simulink model "RecvL4sStEnCtrl"  (R2018b)
settings: Solver=FixedStepDiscrete  StartTime=0.0  StopTime=10.0  FixedStep=0.01  RelTol=1e-3
undefined symbols (not defined in the file or in its folder): data, KeSMSw4SSecRwLtStLgrstOtwdInwdClosePos1_Val, KeSMSw4SSecRwLtStLgrstUpwdDnwdClosePos1_Val, KeSMSw4SSecRwLtStLgrstUpwdDnwdClosePos2_Val, SecRwLtStBkReclnEn_Clear, SecRwLtStBkReclnEn_Set, SecRwLtStFtrstEn_Clear, SecRwLtStFtrstEn_Set, SecRwLtStHdrstFwdBkwdEn_Clear, SecRwLtStHdrstFwdBkwdEn_Set, SecRwLtStHdrstUpwdDnwdEn_Clear, SecRwLtStHdrstUpwdDnwdEn_Set, SecRwLtStLgrstInwdOtwdEn_Clear, SecRwLtStLgrstInwdOtwdEn_Set, SecRwLtStLgrstUpwdDnwdEn_Clear, SecRwLtStLgrstUpwdDnwdEn_Set
libraries: simulink x13
settings Model: Creator=sn2xws  LastModifiedBy=sn2xws
settings DataIOCC: SaveFormat=StructureWithTime
settings OptimizationCC: DefaultParameterBehavior=Inlined  EnhancedBackFolding=on  PassReuseOutputArgsAs=Individual arguments  ZeroExternalMemoryAtStartup=off  ZeroInternalMemoryAtStartup=off  OptimizeBlockOrder=speed  DifferentSizesBufferReuse=on  OptimizationCustomize=off
settings DebuggingCC: ParameterTunabilityLossMsg=error
settings SFSimCC: MATLABDynamicMemAlloc=off
settings RTWCC: SystemTargetFile=autosar.tlc  GenCodeOnly=on  TemplateMakefile=ert_default_tmf  Description=AUTOSAR  GenerateReport=on  IncludeHyperlinkInReport=on  LaunchReport=on  GenerateTraceInfo=on  GenerateTraceReport=on  GenerateTraceReportSl=on  GenerateTraceReportSf=on  GenerateTraceReportEml=on  GenerateCodeMetricsReport=on
settings CodeAppCC: ForceParamTrailComments=on  IgnoreCustomStorageClasses=off  OperatorAnnotations=on  SimulinkDataObjDesc=on  SFDataObjDesc=on  InsertBlockDesc=on
settings STFCustomTargetCC: TargetLangStandard=C99 (ISO)  MultiwordLength=256  ParMdlRefBuildCompliant=on  CompOptLevelCompliant=on  IncludeMdlTerminateFcn=off  CombineOutputUpdateFcns=on  SuppressErrorStatus=on  ERTCustomFileBanners=on  SupportNonFinite=off  SupportComplex=off  SupportContinuousTime=off  SupportNonInlinedSFcns=off  RemoveResetFunc=on  MATLABClassNameForMDSCustomization=Simulink.SoftwareTarget.ERTCustomization  AutosarCompliant=on  UseToolchainInfoCompliant=on  LookupTableObjectStructAxisOrder=2,1,3,4,...  LUTObjectStructOrderEvenSpacing=Size,Table,Breakpoints  SystemTargetFile=autosar.tlc
settings ERTTargetCC: TargetLangStandard=C99 (ISO)  ConcurrentExecutionCompliant=off  IncludeMdlTerminateFcn=off  SuppressErrorStatus=on  SupportNonFinite=off  SupportComplex=off  ModelStepFunctionPrototypeControlCompliant=off  CPPClassGenCompliant=off  AutosarCompliant=on  LookupTableObjectStructAxisOrder=2,1,3,4,...  LUTObjectStructOrderEvenSpacing=Size,Table,Breakpoints  InlinedParameterPlacement=NonHierarchical  ERTCustomFileTemplate=example_file_process.tlc  ERTFilePackagingFormat=Compact

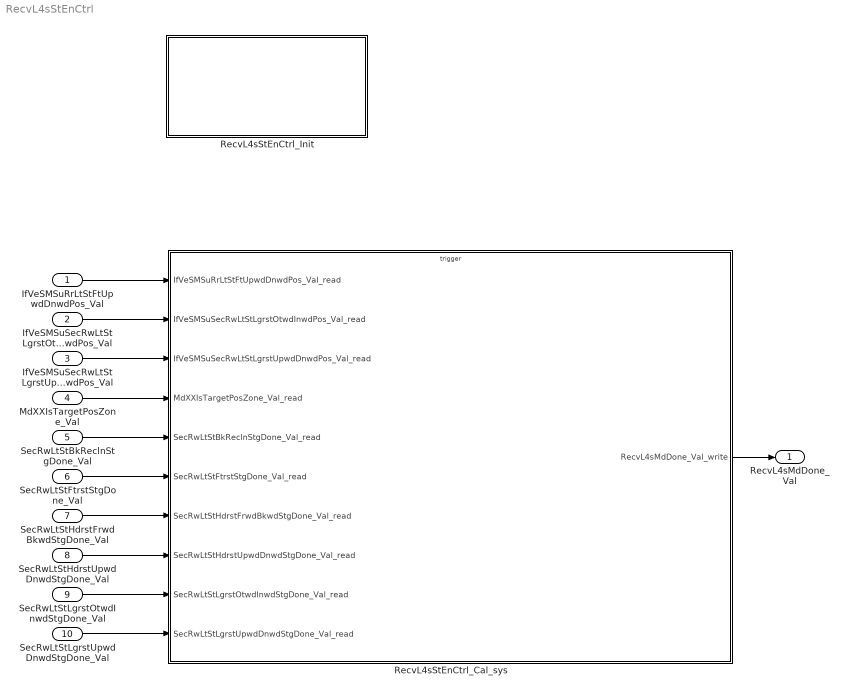
== system RecvL4sStEnCtrl ==
  IfVeSMSuRrLtStFtUpwdDnwdPos_Val : Inport  OutDataTypeStr=uint16  PortDimensions=1
  IfVeSMSuSecRwLtStLgrstOtwdInwdPos_Val : Inport  Port=2  OutDataTypeStr=uint16  PortDimensions=1
  IfVeSMSuSecRwLtStLgrstUpwdDnwdPos_Val : Inport  Port=3  OutDataTypeStr=uint16  PortDimensions=1
  MdXXIsTargetPosZone_Val : Inport  Port=4  OutDataTypeStr=uint32  PortDimensions=1
  SecRwLtStBkReclnStgDone_Val : Inport  Port=5  OutDataTypeStr=boolean  PortDimensions=1
  SecRwLtStFtrstStgDone_Val : Inport  Port=6  OutDataTypeStr=boolean  PortDimensions=1
  SecRwLtStHdrstFrwdBkwdStgDone_Val : Inport  Port=7  OutDataTypeStr=boolean  PortDimensions=1
  SecRwLtStHdrstUpwdDnwdStgDone_Val : Inport  Port=8  OutDataTypeStr=boolean  PortDimensions=1
  SecRwLtStLgrstOtwdInwdStgDone_Val : Inport  Port=9  OutDataTypeStr=boolean  PortDimensions=1
  SecRwLtStLgrstUpwdDnwdStgDone_Val : Inport  Port=10  OutDataTypeStr=boolean  PortDimensions=1
  RecvL4sStEnCtrl_Cal_sys : Subsystem
  RecvL4sStEnCtrl_Init : Subsystem
  RecvL4sMdDone_Val : Outport  OutDataTypeStr=uint8  PortDimensions=1
  wires:
  IfVeSMSuRrLtStFtUpwdDnwdPos_Val/1 -> RecvL4sStEnCtrl_Cal_sys/1(IfVeSMSuRrLtStFtUpwdDnwdPos_Val_read)
  IfVeSMSuSecRwLtStLgrstOtwdInwdPos_Val/1 -> RecvL4sStEnCtrl_Cal_sys/2(IfVeSMSuSecRwLtStLgrstOtwdInwdPos_Val_read)
  IfVeSMSuSecRwLtStLgrstUpwdDnwdPos_Val/1 -> RecvL4sStEnCtrl_Cal_sys/3(IfVeSMSuSecRwLtStLgrstUpwdDnwdPos_Val_read)
  MdXXIsTargetPosZone_Val/1 -> RecvL4sStEnCtrl_Cal_sys/4(MdXXIsTargetPosZone_Val_read)
  SecRwLtStBkReclnStgDone_Val/1 -> RecvL4sStEnCtrl_Cal_sys/5(SecRwLtStBkReclnStgDone_Val_read)
  SecRwLtStFtrstStgDone_Val/1 -> RecvL4sStEnCtrl_Cal_sys/6(SecRwLtStFtrstStgDone_Val_read)
  SecRwLtStHdrstFrwdBkwdStgDone_Val/1 -> RecvL4sStEnCtrl_Cal_sys/7(SecRwLtStHdrstFrwdBkwdStgDone_Val_read)
  SecRwLtStHdrstUpwdDnwdStgDone_Val/1 -> RecvL4sStEnCtrl_Cal_sys/8(SecRwLtStHdrstUpwdDnwdStgDone_Val_read)
  SecRwLtStLgrstOtwdInwdStgDone_Val/1 -> RecvL4sStEnCtrl_Cal_sys/9(SecRwLtStLgrstOtwdInwdStgDone_Val_read)
  SecRwLtStLgrstUpwdDnwdStgDone_Val/1 -> RecvL4sStEnCtrl_Cal_sys/10(SecRwLtStLgrstUpwdDnwdStgDone_Val_read)
  RecvL4sStEnCtrl_Cal_sys/1(RecvL4sMdDone_Val_write) -> RecvL4sMdDone_Val/1

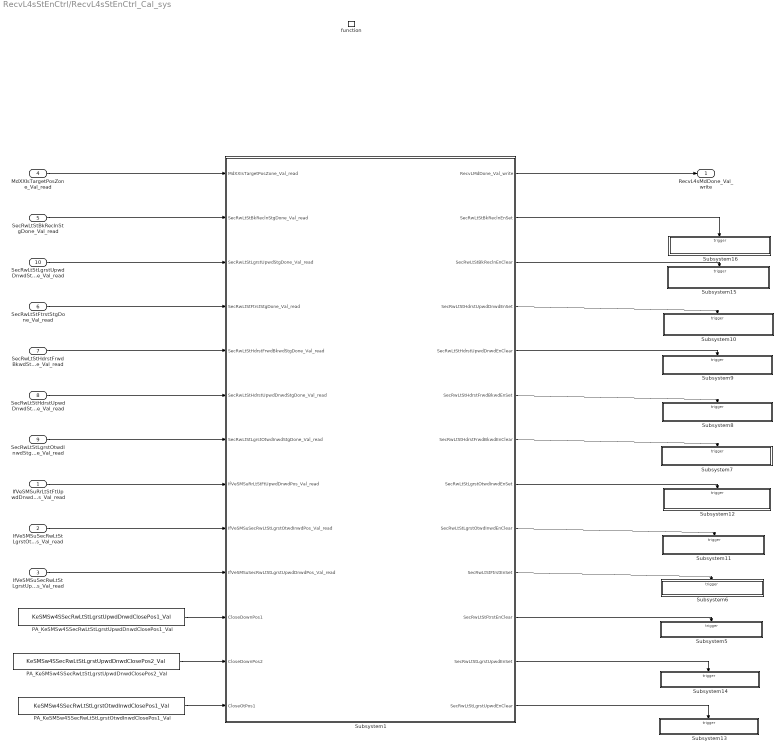
== system RecvL4sStEnCtrl/RecvL4sStEnCtrl_Cal_sys ==
  IfVeSMSuRrLtStFtUpwdDnwdPos_Val_read : Inport
  IfVeSMSuSecRwLtStLgrstOtwdInwdPos_Val_read : Inport  Port=2
  IfVeSMSuSecRwLtStLgrstUpwdDnwdPos_Val_read : Inport  Port=3
  MdXXIsTargetPosZone_Val_read : Inport  Port=4
  SecRwLtStBkReclnStgDone_Val_read : Inport  Port=5
  SecRwLtStFtrstStgDone_Val_read : Inport  Port=6
  SecRwLtStHdrstFrwdBkwdStgDone_Val_read : Inport  Port=7
  SecRwLtStHdrstUpwdDnwdStgDone_Val_read : Inport  Port=8
  SecRwLtStLgrstOtwdInwdStgDone_Val_read : Inport  Port=9
  SecRwLtStLgrstUpwdDnwdStgDone_Val_read : Inport  Port=10
  function : TriggerPort  TriggerType=function-call  IsSimulinkFunction=on  FunctionName=RecvL4sStEnCtrl_Cal  VariantControl=(inherit)
  PA_KeSMSw4SSecRwLtStLgrstOtwdInwdClosePos1_Val : Constant  Value=KeSMSw4SSecRwLtStLgrstOtwdInwdClosePos1_Val
  PA_KeSMSw4SSecRwLtStLgrstUpwdDnwdClosePos1_Val : Constant  Value=KeSMSw4SSecRwLtStLgrstUpwdDnwdClosePos1_Val
  PA_KeSMSw4SSecRwLtStLgrstUpwdDnwdClosePos2_Val : Constant  Value=KeSMSw4SSecRwLtStLgrstUpwdDnwdClosePos2_Val
  Subsystem1 : Subsystem
  Subsystem10 : Subsystem
  Subsystem11 : Subsystem
  Subsystem12 : Subsystem
  Subsystem13 : Subsystem
  Subsystem14 : Subsystem
  Subsystem15 : Subsystem
  Subsystem16 : Subsystem
  Subsystem5 : Subsystem
  Subsystem6 : Subsystem
  Subsystem7 : Subsystem
  Subsystem8 : Subsystem
  Subsystem9 : Subsystem
  RecvL4sMdDone_Val_write : Outport
      settings: EnsureOutportIsVirtual=on
  wires:
  SecRwLtStHdrstFrwdBkwdStgDone_Val_read/1 -> Subsystem1/5(SecRwLtStHdrstFrwdBkwdStgDone_Val_read)
  MdXXIsTargetPosZone_Val_read/1 -> Subsystem1/1(MdXXIsTargetPosZone_Val_read)
  SecRwLtStBkReclnStgDone_Val_read/1 -> Subsystem1/2(SecRwLtStBkReclnStgDone_Val_read)
  SecRwLtStLgrstUpwdDnwdStgDone_Val_read/1 -> Subsystem1/3(SecRwLtStLgrstUpwdStgDone_Val_read)
  SecRwLtStFtrstStgDone_Val_read/1 -> Subsystem1/4(SecRwLtStFtrstStgDone_Val_read)
  SecRwLtStHdrstUpwdDnwdStgDone_Val_read/1 -> Subsystem1/6(SecRwLtStHdrstUpwdDnwdStgDone_Val_read)
  SecRwLtStLgrstOtwdInwdStgDone_Val_read/1 -> Subsystem1/7(SecRwLtStLgrstOtwdInwdStgDone_Val_read)
  IfVeSMSuRrLtStFtUpwdDnwdPos_Val_read/1 -> Subsystem1/8(IfVeSMSuRrLtStFtUpwdDnwdPos_Val_read)
  IfVeSMSuSecRwLtStLgrstOtwdInwdPos_Val_read/1 -> Subsystem1/9(IfVeSMSuSecRwLtStLgrstOtwdInwdPos_Val_read)
  IfVeSMSuSecRwLtStLgrstUpwdDnwdPos_Val_read/1 -> Subsystem1/10(IfVeSMSuSecRwLtStLgrstUpwdDnwdPos_Val_read)
  PA_KeSMSw4SSecRwLtStLgrstOtwdInwdClosePos1_Val/1 -> Subsystem1/13(CloseOtPos1)
  PA_KeSMSw4SSecRwLtStLgrstUpwdDnwdClosePos1_Val/1 -> Subsystem1/11(CloseDownPos1)
  PA_KeSMSw4SSecRwLtStLgrstUpwdDnwdClosePos2_Val/1 -> Subsystem1/12(CloseDownPos2)
  Subsystem1/1(RecvLMdDone_Val_write) -> RecvL4sMdDone_Val_write/1
  Subsystem1/5(SecRwLtStHdrstUpwdDnwdEnClear) -> Subsystem9/Trigger
  Subsystem1/3(SecRwLtStBkReclnEnClear) -> Subsystem15/Trigger
  Subsystem1/9(SecRwLtStLgrstOtwdInwdEnClear) -> Subsystem11/Trigger
  Subsystem1/8(SecRwLtStLgrstOtwdInwdEnSet) -> Subsystem12/Trigger
  Subsystem1/6(SecRwLtStHdrstFrwdBkwdEnSet) -> Subsystem8/Trigger
  Subsystem1/12(SecRwLtStLgrstUpwdEnSet) -> Subsystem14/Trigger
  Subsystem1/13(SecRwLtStLgrstUpwdEnClear) -> Subsystem13/Trigger
  Subsystem1/2(SecRwLtStBkReclnEnSet) -> Subsystem16/Trigger
  Subsystem1/11(SecRwLtStFtrstEnClear) -> Subsystem5/Trigger
  Subsystem1/7(SecRwLtStHdrstFrwdBkwdEnClear) -> Subsystem7/Trigger
  Subsystem1/10(SecRwLtStFtrstEnSet) -> Subsystem6/Trigger
  Subsystem1/4(SecRwLtStHdrstUpwdDnwdEnSet) -> Subsystem10/Trigger

== system RecvL4sStEnCtrl/RecvL4sStEnCtrl_Init ==
  Event Listener : EventListener  EventName=reset

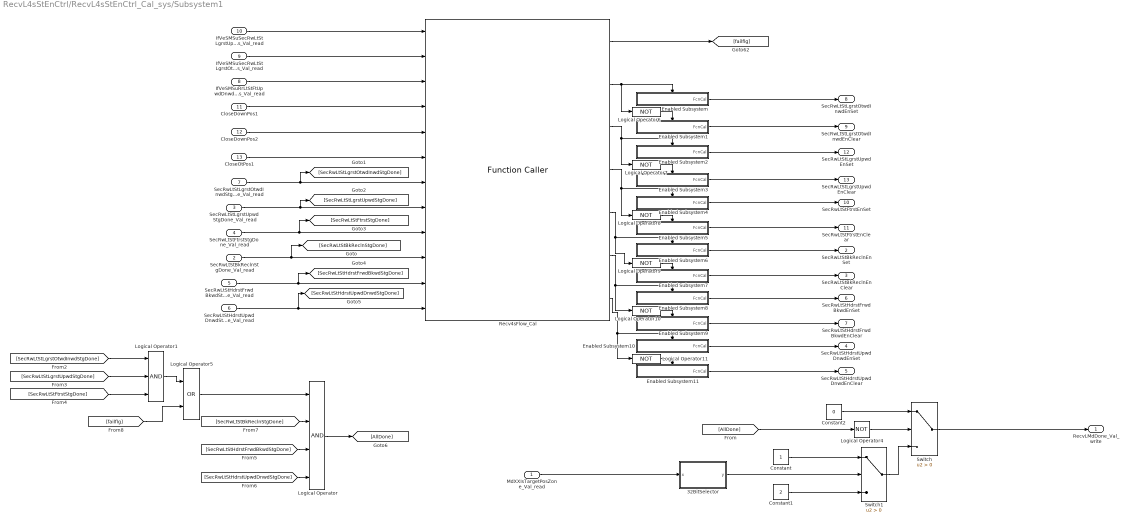
== system RecvL4sStEnCtrl/RecvL4sStEnCtrl_Cal_sys/Subsystem1 ==
  MdXXIsTargetPosZone_Val_read : Inport
  SecRwLtStBkReclnStgDone_Val_read : Inport  Port=2
  SecRwLtStLgrstUpwdStgDone_Val_read : Inport  Port=3
  SecRwLtStFtrstStgDone_Val_read : Inport  Port=4
  SecRwLtStHdrstFrwdBkwdStgDone_Val_read : Inport  Port=5
  SecRwLtStHdrstUpwdDnwdStgDone_Val_read : Inport  Port=6
  SecRwLtStLgrstOtwdInwdStgDone_Val_read : Inport  Port=7
  IfVeSMSuRrLtStFtUpwdDnwdPos_Val_read : Inport  Port=8
  IfVeSMSuSecRwLtStLgrstOtwdInwdPos_Val_read : Inport  Port=9
  IfVeSMSuSecRwLtStLgrstUpwdDnwdPos_Val_read : Inport  Port=10
  CloseDownPos1 : Inport  Port=11
  CloseDownPos2 : Inport  Port=12
  CloseOtPos1 : Inport  Port=13
  32BitSelector : Subsystem  mask(32 Bit Selector){BitNum=10}
      mask prompts: BitNum "Select Bit Number"
      mask help: Allows selection of a particular bit (0-31) out of a packed word up to 32 bits long. Output will be true if the bit number selected via the mask parameter is equal to one.
      mask TypeOptions BitNum: 0 | 1 | 2 | 3 | 4 | 5 | 6 | 7 | 8 | 9 | 10 | 11 | 12 | 13 | 14 | 15 | 16 | 17 | 18 | 19 | 20 | 21 | 22 | 23 | 24 | 25 | 26 | 27 | 28 | 29 | 30 | 31
      mask Display:
      | text(0.5, 0.8,'BIT','horizontalAlignment','center')
      | text(0.5, 0.5,'SELECTOR','horizontalAlignment','center')
      | text(0.5, 0.2,['-- Bit ',char(get_param(gcb,'BitNum')),' --'],'horizontalAlignment','center')
  Constant : Constant  OutDataTypeStr=uint8
  Constant1 : Constant  Value=2  OutDataTypeStr=uint8
  Constant2 : Constant  Value=0  OutDataTypeStr=uint8
  Enabled Subsystem : Subsystem  TreatAsAtomicUnit=on
  Enabled Subsystem1 : Subsystem  TreatAsAtomicUnit=on
  Enabled Subsystem10 : Subsystem  TreatAsAtomicUnit=on
  Enabled Subsystem11 : Subsystem  TreatAsAtomicUnit=on
  Enabled Subsystem2 : Subsystem  TreatAsAtomicUnit=on
  Enabled Subsystem3 : Subsystem  TreatAsAtomicUnit=on
  Enabled Subsystem4 : Subsystem  TreatAsAtomicUnit=on
  Enabled Subsystem5 : Subsystem  TreatAsAtomicUnit=on
  Enabled Subsystem6 : Subsystem  TreatAsAtomicUnit=on
  Enabled Subsystem7 : Subsystem  TreatAsAtomicUnit=on
  Enabled Subsystem8 : Subsystem  TreatAsAtomicUnit=on
  Enabled Subsystem9 : Subsystem  TreatAsAtomicUnit=on
  Logical Operator : Logic  Inputs=4  AllPortsSameDT=off  OutDataTypeStr=boolean
  Logical Operator1 : Logic  Inputs=3  AllPortsSameDT=off  OutDataTypeStr=boolean
  Logical Operator{4,6..11} (7 alike) : Logic  Operator=NOT  AllPortsSameDT=off  OutDataTypeStr=boolean
  Logical Operator5 : Logic  Operator=OR  AllPortsSameDT=off  OutDataTypeStr=boolean
  Recv4sFlow_Cal : FunctionCaller  FunctionPrototype=[Failflg,LgrstInwdOtwdEn,LgrstUpwdDnwdEn,FtrstEn,BkReclnEn,HdrstFrwdBkwdEn,HdrstUpwdDnwdEn] = Recv4sFlow_Cal(LgrstUpwdDnwdPos,LgrstOtwdInwdPos,FtUpwdDnwdPos,CloseDnwdPos1,CloseDnwdPos2,CloseOtwdPos1,LgrstInwdStgDone,LgrstUpwdStgDone,FtrstStgDone,BkReclnStgDone,HdrstFwdBkwdStgDone,HdrstupwdDnwdStgDone)  InputArgumentSpecifications=uint16(1), uint16(1), uint16(1), uint16(1), uint16(1), uint16(1), boolean(true), boolean(true), boolean(true), boolean(true), boolean(true), boolean(true)  OutputArgumentSpecifications=boolean(true), boolean(true), boolean(true), boolean(true), boolean(true), boolean(true), boolean(true)
  Switch : Switch  Criteria=u2 > Threshold
  Switch1 : Switch  Criteria=u2 > Threshold
  RecvLMdDone_Val_write : Outport
      settings: EnsureOutportIsVirtual=on
  SecRwLtStBkReclnEnSet : Outport  Port=2
  SecRwLtStBkReclnEnClear : Outport  Port=3
  SecRwLtStHdrstUpwdDnwdEnSet : Outport  Port=4
  SecRwLtStHdrstUpwdDnwdEnClear : Outport  Port=5
  SecRwLtStHdrstFrwdBkwdEnSet : Outport  Port=6
  SecRwLtStHdrstFrwdBkwdEnClear : Outport  Port=7
  SecRwLtStLgrstOtwdInwdEnSet : Outport  Port=8
  SecRwLtStLgrstOtwdInwdEnClear : Outport  Port=9
  SecRwLtStFtrstEnSet : Outport  Port=10
  SecRwLtStFtrstEnClear : Outport  Port=11
  SecRwLtStLgrstUpwdEnSet : Outport  Port=12
  SecRwLtStLgrstUpwdEnClear : Outport  Port=13
  wires:
  SecRwLtStLgrstOtwdInwdStgDone_Val_read/1 -> Recv4sFlow_Cal/7, [SecRwLtStLgrstOtwdInwdStgDone]
  Recv4sFlow_Cal/1 -> [failflg]
  CloseDownPos2/1 -> Recv4sFlow_Cal/5
  SecRwLtStHdrstUpwdDnwdStgDone_Val_read/1 -> [SecRwLtStHdrstUpwdDnwdStgDone], Recv4sFlow_Cal/12
  IfVeSMSuRrLtStFtUpwdDnwdPos_Val_read/1 -> Recv4sFlow_Cal/3
  CloseDownPos1/1 -> Recv4sFlow_Cal/4
  SecRwLtStHdrstFrwdBkwdStgDone_Val_read/1 -> [SecRwLtStHdrstFrwdBkwdStgDone], Recv4sFlow_Cal/11
  CloseOtPos1/1 -> Recv4sFlow_Cal/6
  IfVeSMSuSecRwLtStLgrstUpwdDnwdPos_Val_read/1 -> Recv4sFlow_Cal/1
  SecRwLtStBkReclnStgDone_Val_read/1 -> [SecRwLtStBkReclnStgDone], Recv4sFlow_Cal/10
  IfVeSMSuSecRwLtStLgrstOtwdInwdPos_Val_read/1 -> Recv4sFlow_Cal/2
  SecRwLtStLgrstUpwdStgDone_Val_read/1 -> Recv4sFlow_Cal/8, [SecRwLtStLgrstUpwdStgDone]
  Switch/1 -> RecvLMdDone_Val_write/1
  MdXXIsTargetPosZone_Val_read/1 -> 32BitSelector/1(x)
  Switch1/1 -> Switch/3
  SecRwLtStFtrstStgDone_Val_read/1 -> [SecRwLtStFtrstStgDone], Recv4sFlow_Cal/9
  Logical Operator5/1 -> Logical Operator/1
  [SecRwLtStFtrstStgDone] -> Logical Operator1/3
  Logical Operator1/1 -> Logical Operator5/1
  [SecRwLtStLgrstOtwdInwdStgDone] -> Logical Operator1/1
  [failflg] -> Logical Operator5/2
  [SecRwLtStLgrstUpwdStgDone] -> Logical Operator1/2
  [SecRwLtStHdrstUpwdDnwdStgDone] -> Logical Operator/4
  [SecRwLtStHdrstFrwdBkwdStgDone] -> Logical Operator/3
  [SecRwLtStBkReclnStgDone] -> Logical Operator/2
  Logical Operator/1 -> [AllDone]
  Enabled Subsystem6/1(FcnCal) -> SecRwLtStBkReclnEnSet/1
  Enabled Subsystem7/1(FcnCal) -> SecRwLtStBkReclnEnClear/1
  Enabled Subsystem2/1(FcnCal) -> SecRwLtStLgrstUpwdEnSet/1
  Enabled Subsystem3/1(FcnCal) -> SecRwLtStLgrstUpwdEnClear/1
  Enabled Subsystem10/1(FcnCal) -> SecRwLtStHdrstUpwdDnwdEnSet/1
  Enabled Subsystem11/1(FcnCal) -> SecRwLtStHdrstUpwdDnwdEnClear/1
  Enabled Subsystem8/1(FcnCal) -> SecRwLtStHdrstFrwdBkwdEnSet/1
  Enabled Subsystem9/1(FcnCal) -> SecRwLtStHdrstFrwdBkwdEnClear/1
  Enabled Subsystem/1(FcnCal) -> SecRwLtStLgrstOtwdInwdEnSet/1
  Enabled Subsystem1/1(FcnCal) -> SecRwLtStLgrstOtwdInwdEnClear/1
  Recv4sFlow_Cal/2 -> Logical Operator6/1, Enabled Subsystem/Enable
  Logical Operator6/1 -> Enabled Subsystem1/Enable
  Logical Operator7/1 -> Enabled Subsystem3/Enable
  Recv4sFlow_Cal/3 -> Logical Operator7/1, Enabled Subsystem2/Enable
  Recv4sFlow_Cal/4 -> Enabled Subsystem4/Enable, Logical Operator8/1
  Logical Operator8/1 -> Enabled Subsystem5/Enable
  Enabled Subsystem4/1(FcnCal) -> SecRwLtStFtrstEnSet/1
  Enabled Subsystem5/1(FcnCal) -> SecRwLtStFtrstEnClear/1
  Logical Operator9/1 -> Enabled Subsystem7/Enable
  Recv4sFlow_Cal/5 -> Enabled Subsystem6/Enable, Logical Operator9/1
  Recv4sFlow_Cal/6 -> Enabled Subsystem8/Enable, Logical Operator10/1
  Logical Operator10/1 -> Enabled Subsystem9/Enable
  Logical Operator11/1 -> Enabled Subsystem11/Enable
  Recv4sFlow_Cal/7 -> Logical Operator11/1, Enabled Subsystem10/Enable
  Constant2/1 -> Switch/1
  Constant1/1 -> Switch1/3
  Constant/1 -> Switch1/1
  [AllDone] -> Logical Operator4/1
  Logical Operator4/1 -> Switch/2
  32BitSelector/1(y) -> Switch1/2

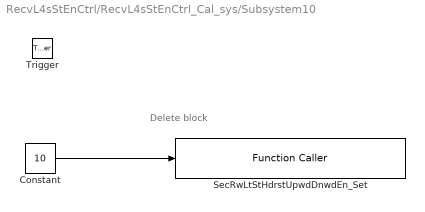
== system RecvL4sStEnCtrl/RecvL4sStEnCtrl_Cal_sys/Subsystem10 ==
  note: Delete block
  Trigger : TriggerPort  TriggerType=function-call  VariantControl=Variant  PortDimensions=1
  Constant : Constant  Value=10  OutDataTypeStr=uint8
  SecRwLtStHdrstUpwdDnwdEn_Set : FunctionCaller  FunctionPrototype=SecRwLtStHdrstUpwdDnwdEn_Set(data)  InputArgumentSpecifications=uint8(1)
  wires:
  Constant/1 -> SecRwLtStHdrstUpwdDnwdEn_Set/1

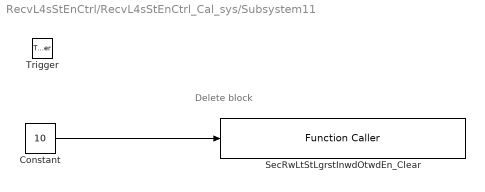
== system RecvL4sStEnCtrl/RecvL4sStEnCtrl_Cal_sys/Subsystem11 ==
  note: Delete block
  Trigger : TriggerPort  TriggerType=function-call  VariantControl=Variant  PortDimensions=1
  Constant : Constant  Value=10  OutDataTypeStr=uint8
  SecRwLtStLgrstInwdOtwdEn_Clear : FunctionCaller  FunctionPrototype=SecRwLtStLgrstInwdOtwdEn_Clear(data)  InputArgumentSpecifications=uint8(1)
  wires:
  Constant/1 -> SecRwLtStLgrstInwdOtwdEn_Clear/1

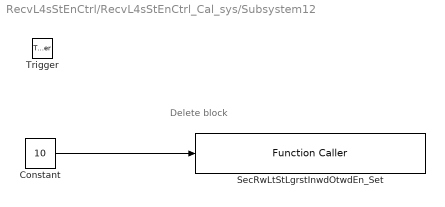
== system RecvL4sStEnCtrl/RecvL4sStEnCtrl_Cal_sys/Subsystem12 ==
  note: Delete block
  Trigger : TriggerPort  TriggerType=function-call  VariantControl=Variant  PortDimensions=1
  Constant : Constant  Value=10  OutDataTypeStr=uint8
  SecRwLtStLgrstInwdOtwdEn_Set : FunctionCaller  FunctionPrototype=SecRwLtStLgrstInwdOtwdEn_Set(data)  InputArgumentSpecifications=uint8(1)
  wires:
  Constant/1 -> SecRwLtStLgrstInwdOtwdEn_Set/1

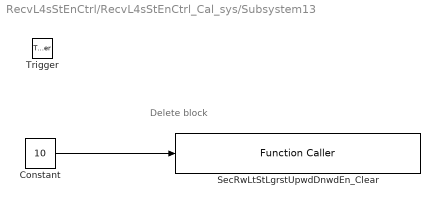
== system RecvL4sStEnCtrl/RecvL4sStEnCtrl_Cal_sys/Subsystem13 ==
  note: Delete block
  Trigger : TriggerPort  TriggerType=function-call  VariantControl=Variant  PortDimensions=1
  Constant : Constant  Value=10  OutDataTypeStr=uint8
  SecRwLtStLgrstUpwdDnwdEn_Clear : FunctionCaller  FunctionPrototype=SecRwLtStLgrstUpwdDnwdEn_Clear(data)  InputArgumentSpecifications=uint8(1)
  wires:
  Constant/1 -> SecRwLtStLgrstUpwdDnwdEn_Clear/1

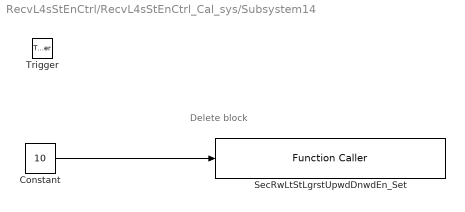
== system RecvL4sStEnCtrl/RecvL4sStEnCtrl_Cal_sys/Subsystem14 ==
  note: Delete block
  Trigger : TriggerPort  TriggerType=function-call  VariantControl=Variant  PortDimensions=1
  Constant : Constant  Value=10  OutDataTypeStr=uint8
  SecRwLtStLgrstUpwdDnwdEn_Set : FunctionCaller  FunctionPrototype=SecRwLtStLgrstUpwdDnwdEn_Set(data)  InputArgumentSpecifications=uint8(1)
  wires:
  Constant/1 -> SecRwLtStLgrstUpwdDnwdEn_Set/1

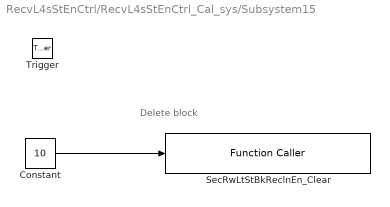
== system RecvL4sStEnCtrl/RecvL4sStEnCtrl_Cal_sys/Subsystem15 ==
  note: Delete block
  Trigger : TriggerPort  TriggerType=function-call  VariantControl=Variant  PortDimensions=1
  Constant : Constant  Value=10  OutDataTypeStr=uint8
  SecRwLtStBkReclnEn_Clear : FunctionCaller  FunctionPrototype=SecRwLtStBkReclnEn_Clear(data)  InputArgumentSpecifications=uint8(1)
  wires:
  Constant/1 -> SecRwLtStBkReclnEn_Clear/1

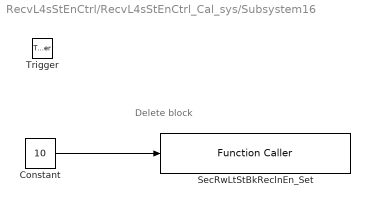
== system RecvL4sStEnCtrl/RecvL4sStEnCtrl_Cal_sys/Subsystem16 ==
  note: Delete block
  Trigger : TriggerPort  TriggerType=function-call  VariantControl=Variant  PortDimensions=1
  Constant : Constant  Value=10  OutDataTypeStr=uint8
  SecRwLtStBkReclnEn_Set : FunctionCaller  FunctionPrototype=SecRwLtStBkReclnEn_Set(data)  InputArgumentSpecifications=uint8(1)
  wires:
  Constant/1 -> SecRwLtStBkReclnEn_Set/1

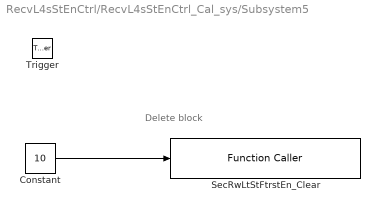
== system RecvL4sStEnCtrl/RecvL4sStEnCtrl_Cal_sys/Subsystem5 ==
  note: Delete block
  Trigger : TriggerPort  TriggerType=function-call  VariantControl=Variant  PortDimensions=1
  Constant : Constant  Value=10  OutDataTypeStr=uint8
  SecRwLtStFtrstEn_Clear : FunctionCaller  FunctionPrototype=SecRwLtStFtrstEn_Clear(data)  InputArgumentSpecifications=uint8(1)
  wires:
  Constant/1 -> SecRwLtStFtrstEn_Clear/1

== system RecvL4sStEnCtrl/RecvL4sStEnCtrl_Cal_sys/Subsystem6 ==
  note: Delete block
  Trigger : TriggerPort  TriggerType=function-call  VariantControl=Variant  PortDimensions=1
  Constant : Constant  Value=10  OutDataTypeStr=uint8
  SecRwLtStFtrstEn_Set : FunctionCaller  FunctionPrototype=SecRwLtStFtrstEn_Set(data)  InputArgumentSpecifications=uint8(1)
  wires:
  Constant/1 -> SecRwLtStFtrstEn_Set/1

== system RecvL4sStEnCtrl/RecvL4sStEnCtrl_Cal_sys/Subsystem7 ==
  note: Delete block
  Trigger : TriggerPort  TriggerType=function-call  VariantControl=Variant  PortDimensions=1
  Constant : Constant  Value=10  OutDataTypeStr=uint8
  SecRwLtStHdrstFwdBkwdEn_Clear : FunctionCaller  FunctionPrototype=SecRwLtStHdrstFwdBkwdEn_Clear(data)  InputArgumentSpecifications=uint8(1)
  wires:
  Constant/1 -> SecRwLtStHdrstFwdBkwdEn_Clear/1

== system RecvL4sStEnCtrl/RecvL4sStEnCtrl_Cal_sys/Subsystem8 ==
  note: Delete block
  Trigger : TriggerPort  TriggerType=function-call  VariantControl=Variant  PortDimensions=1
  Constant : Constant  Value=10  OutDataTypeStr=uint8
  SecRwLtStHdrstFwdBkwdEn_Set : FunctionCaller  FunctionPrototype=SecRwLtStHdrstFwdBkwdEn_Set(data)  InputArgumentSpecifications=uint8(1)
  wires:
  Constant/1 -> SecRwLtStHdrstFwdBkwdEn_Set/1

== system RecvL4sStEnCtrl/RecvL4sStEnCtrl_Cal_sys/Subsystem9 ==
  note: Delete block
  Trigger : TriggerPort  TriggerType=function-call  VariantControl=Variant  PortDimensions=1
  Constant : Constant  Value=10  OutDataTypeStr=uint8
  SecRwLtStHdrstUpwdDnwdEn_Clear : FunctionCaller  FunctionPrototype=SecRwLtStHdrstUpwdDnwdEn_Clear(data)  InputArgumentSpecifications=uint8(1)
  wires:
  Constant/1 -> SecRwLtStHdrstUpwdDnwdEn_Clear/1

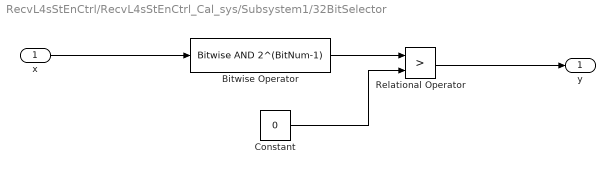
== system RecvL4sStEnCtrl/RecvL4sStEnCtrl_Cal_sys/Subsystem1/32BitSelector ==
  x : Inport
  Bitwise Operator : simulink/Logic and Bit Operations/Bitwise Operator  logicop=AND  UseBitMask=on  BitMask=2^(BitNum-1)  BitMaskRealWorld=Stored Integer
  Constant : Constant  Value=0  OutDataTypeStr=uint32
  Relational Operator : RelationalOperator  Operator=>  OutDataTypeStr=boolean  RndMeth=Simplest
  y : Outport
  wires:
  Relational Operator/1 -> y/1
  Constant/1 -> Relational Operator/2
  x/1 -> Bitwise Operator/1
  Bitwise Operator/1 -> Relational Operator/1

== system RecvL4sStEnCtrl/RecvL4sStEnCtrl_Cal_sys/Subsystem1/Enabled Subsystem ==
  Enable : EnablePort
  Function-Call Generator : simulink/Ports & Subsystems/Function-Call Generator  sample_time=-1  numberOfIterations=1
  FcnCal : Outport
  wires:
  Function-Call Generator/1 -> FcnCal/1

== system RecvL4sStEnCtrl/RecvL4sStEnCtrl_Cal_sys/Subsystem1/Enabled Subsystem1 ==
  Enable : EnablePort
  Function-Call Generator : simulink/Ports & Subsystems/Function-Call Generator  sample_time=-1  numberOfIterations=1
  FcnCal : Outport
  wires:
  Function-Call Generator/1 -> FcnCal/1

== system RecvL4sStEnCtrl/RecvL4sStEnCtrl_Cal_sys/Subsystem1/Enabled Subsystem10 ==
  Enable : EnablePort
  Function-Call Generator : simulink/Ports & Subsystems/Function-Call Generator  sample_time=-1  numberOfIterations=1
  FcnCal : Outport
  wires:
  Function-Call Generator/1 -> FcnCal/1

== system RecvL4sStEnCtrl/RecvL4sStEnCtrl_Cal_sys/Subsystem1/Enabled Subsystem11 ==
  Enable : EnablePort
  Function-Call Generator : simulink/Ports & Subsystems/Function-Call Generator  sample_time=-1  numberOfIterations=1
  FcnCal : Outport
  wires:
  Function-Call Generator/1 -> FcnCal/1

== system RecvL4sStEnCtrl/RecvL4sStEnCtrl_Cal_sys/Subsystem1/Enabled Subsystem2 ==
  Enable : EnablePort
  Function-Call Generator : simulink/Ports & Subsystems/Function-Call Generator  sample_time=-1  numberOfIterations=1
  FcnCal : Outport
  wires:
  Function-Call Generator/1 -> FcnCal/1

== system RecvL4sStEnCtrl/RecvL4sStEnCtrl_Cal_sys/Subsystem1/Enabled Subsystem3 ==
  Enable : EnablePort
  Function-Call Generator : simulink/Ports & Subsystems/Function-Call Generator  sample_time=-1  numberOfIterations=1
  FcnCal : Outport
  wires:
  Function-Call Generator/1 -> FcnCal/1

== system RecvL4sStEnCtrl/RecvL4sStEnCtrl_Cal_sys/Subsystem1/Enabled Subsystem4 ==
  Enable : EnablePort
  Function-Call Generator : simulink/Ports & Subsystems/Function-Call Generator  sample_time=-1  numberOfIterations=1
  FcnCal : Outport
  wires:
  Function-Call Generator/1 -> FcnCal/1

== system RecvL4sStEnCtrl/RecvL4sStEnCtrl_Cal_sys/Subsystem1/Enabled Subsystem5 ==
  Enable : EnablePort
  Function-Call Generator : simulink/Ports & Subsystems/Function-Call Generator  sample_time=-1  numberOfIterations=1
  FcnCal : Outport
  wires:
  Function-Call Generator/1 -> FcnCal/1

== system RecvL4sStEnCtrl/RecvL4sStEnCtrl_Cal_sys/Subsystem1/Enabled Subsystem6 ==
  Enable : EnablePort
  Function-Call Generator : simulink/Ports & Subsystems/Function-Call Generator  sample_time=-1  numberOfIterations=1
  FcnCal : Outport
  wires:
  Function-Call Generator/1 -> FcnCal/1

== system RecvL4sStEnCtrl/RecvL4sStEnCtrl_Cal_sys/Subsystem1/Enabled Subsystem7 ==
  Enable : EnablePort
  Function-Call Generator : simulink/Ports & Subsystems/Function-Call Generator  sample_time=-1  numberOfIterations=1
  FcnCal : Outport
  wires:
  Function-Call Generator/1 -> FcnCal/1

== system RecvL4sStEnCtrl/RecvL4sStEnCtrl_Cal_sys/Subsystem1/Enabled Subsystem8 ==
  Enable : EnablePort
  Function-Call Generator : simulink/Ports & Subsystems/Function-Call Generator  sample_time=-1  numberOfIterations=1
  FcnCal : Outport
  wires:
  Function-Call Generator/1 -> FcnCal/1

== system RecvL4sStEnCtrl/RecvL4sStEnCtrl_Cal_sys/Subsystem1/Enabled Subsystem9 ==
  Enable : EnablePort
  Function-Call Generator : simulink/Ports & Subsystems/Function-Call Generator  sample_time=-1  numberOfIterations=1
  FcnCal : Outport
  wires:
  Function-Call Generator/1 -> FcnCal/1
